simulink model "reference_model"  (R2023b)
settings: Solver=VariableStepAuto  StartTime=0.0  StopTime=10.0  RelTol=1e-3
values from neighbouring files (symbols this model uses):
  w = 7    [CA3_params.m]    (also in CA3_params_integral.m; CA3_params_yp.m)
  xi = 0.6    [CA3_params.m]    (also in CA3_params_integral.m; CA3_params_yp.m)
settings Model: Creator=john  LastModifiedBy=john

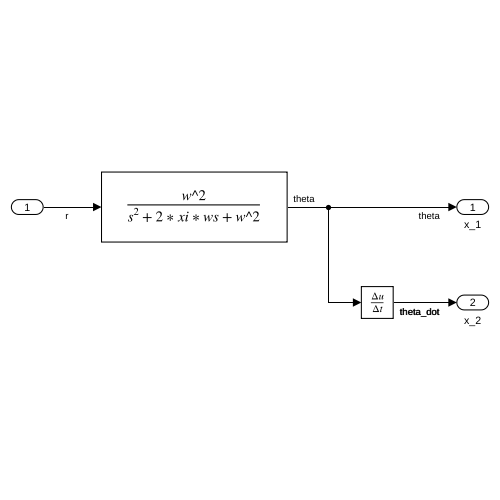
[thumbnail: Simulink's stored preview of the top-level diagram]
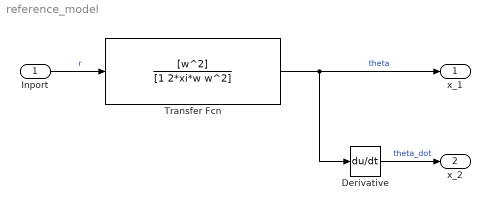
== system reference_model ==
  Inport : Inport
  Derivative : Derivative
  Transfer Fcn : TransferFcn  Numerator=[w^2]  Denominator=[1 2*xi*w w^2]
  x_1 : Outport
  x_2 : Outport  Port=2
  wires:
  Inport/1 -> Transfer Fcn/1  "r"
  Transfer Fcn/1 -> x_1/1, Derivative/1  "theta"
  Derivative/1 -> x_2/1  "theta_dot"
